simulink model "zad2"  (R2020b)
settings: Solver=FixedStepDiscrete  StartTime=0.0  StopTime=0.0  RelTol=1e-3
libraries: CPOiS_SourcesSinks x11, CPOiS_DataManipulation_DataTypeConversion x4, CPOiS_LinearTransforms x3, CPOiS_HistogramOperations x3, CPOiS_Filters x2, CPOiS_General x1
settings Model: Creator=jrybarz  LastModifiedBy=jrybarz

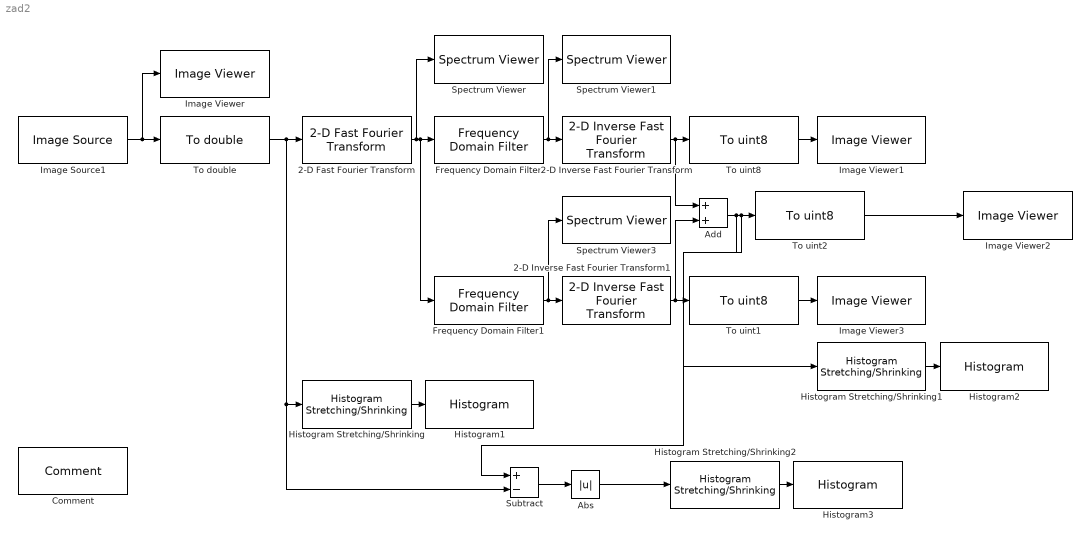
== system zad2 ==
  2-D Fast Fourier Transform : CPOiS_LinearTransforms/2-D Fast Fourier Transform
      settings: SourceProductName=CPOiS - Digital image and signal processing
  2-D Inverse Fast Fourier Transform : CPOiS_LinearTransforms/2-D Inverse Fast  Fourier Transform
      settings: SourceProductName=CPOiS - Digital image and signal processing
  2-D Inverse Fast Fourier Transform1 : CPOiS_LinearTransforms/2-D Inverse Fast  Fourier Transform
      settings: SourceProductName=CPOiS - Digital image and signal processing
  Abs : Abs
  Add : Sum
  Comment : CPOiS_General/Comment
      settings: SourceProductName=CPOiS - Digital image and signal processing
  Frequency Domain Filter : CPOiS_Filters/Frequency Domain Filter  filtertype=Low-pass Filter  radius=10
      settings: SourceProductName=CPOiS - Digital image and signal processing
  Frequency Domain Filter1 : CPOiS_Filters/Frequency Domain Filter  filtertype=High-pass Filter  radius=10
      settings: SourceProductName=CPOiS - Digital image and signal processing
  Histogram Stretching/Shrinking : CPOiS_HistogramOperations/Histogram Stretching//Shrinking  minimum=0  maximum=255
      settings: SourceProductName=CPOiS - Digital image and signal processing
  Histogram Stretching/Shrinking1 : CPOiS_HistogramOperations/Histogram Stretching//Shrinking  minimum=0  maximum=255
      settings: SourceProductName=CPOiS - Digital image and signal processing
  Histogram Stretching/Shrinking2 : CPOiS_HistogramOperations/Histogram Stretching//Shrinking  minimum=0  maximum=255
      settings: SourceProductName=CPOiS - Digital image and signal processing
  Histogram1 : CPOiS_SourcesSinks/Histogram
      settings: SourceProductName=CPOiS - Digital image and signal processing
  Histogram2 : CPOiS_SourcesSinks/Histogram
      settings: SourceProductName=CPOiS - Digital image and signal processing
  Histogram3 : CPOiS_SourcesSinks/Histogram
      settings: SourceProductName=CPOiS - Digital image and signal processing
  Image Source1 : CPOiS_SourcesSinks/Image Source  FileSelection=concordorthophoto.png
      settings: SourceProductName=CPOiS - Digital image and signal processing
  Image Viewer{,1..3} (4 alike) : CPOiS_SourcesSinks/Image Viewer
      settings: SourceProductName=CPOiS - Digital image and signal processing
  Spectrum Viewer : CPOiS_SourcesSinks/Spectrum Viewer
      settings: SourceProductName=CPOiS - Digital image and signal processing
  Spectrum Viewer1 : CPOiS_SourcesSinks/Spectrum Viewer
      settings: SourceProductName=CPOiS - Digital image and signal processing
  Spectrum Viewer3 : CPOiS_SourcesSinks/Spectrum Viewer
      settings: SourceProductName=CPOiS - Digital image and signal processing
  Subtract : Sum  Inputs=+-
  To double : CPOiS_DataManipulation_DataTypeConversion/To double
      settings: SourceProductName=CPOiS - Digital image and signal processing
  To uint1 : CPOiS_DataManipulation_DataTypeConversion/To uint8
      settings: SourceProductName=CPOiS - Digital image and signal processing
  To uint2 : CPOiS_DataManipulation_DataTypeConversion/To uint8
      settings: SourceProductName=CPOiS - Digital image and signal processing
  To uint8 : CPOiS_DataManipulation_DataTypeConversion/To uint8
      settings: SourceProductName=CPOiS - Digital image and signal processing
  wires:
  2-D Inverse Fast Fourier Transform/1 -> Add/1, To uint8/1
  Image Source1/1 -> Image Viewer/1, To double/1
  To uint8/1 -> Image Viewer1/1
  2-D Fast Fourier Transform/1 -> Spectrum Viewer/1, Frequency Domain Filter1/1, Frequency Domain Filter/1
  Frequency Domain Filter/1 -> Spectrum Viewer1/1, 2-D Inverse Fast Fourier Transform/1
  Frequency Domain Filter1/1 -> Spectrum Viewer3/1, 2-D Inverse Fast Fourier Transform1/1
  2-D Inverse Fast Fourier Transform1/1 -> Add/2, To uint1/1
  To uint1/1 -> Image Viewer3/1
  To uint2/1 -> Image Viewer2/1
  Histogram Stretching/Shrinking/1 -> Histogram1/1
  Histogram Stretching/Shrinking1/1 -> Histogram2/1
  Histogram Stretching/Shrinking2/1 -> Histogram3/1
  Add/1 -> Histogram Stretching/Shrinking1/1, Subtract/1, To uint2/1
  To double/1 -> Subtract/2, Histogram Stretching/Shrinking/1, 2-D Fast Fourier Transform/1
  Subtract/1 -> Abs/1
  Abs/1 -> Histogram Stretching/Shrinking2/1
